simulink model "test2"  (R2019b)
settings: Solver=VariableStepAuto  StartTime=0.0  StopTime=10.0  RelTol=1e-3
libraries: simulink x1
settings Model: Creator=yango  LastModifiedBy=yango

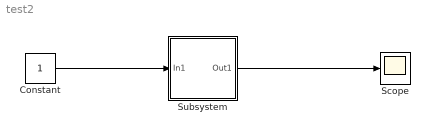
== system test2 ==
  Constant : Constant
  Scope : Scope
  Subsystem : Subsystem
  wires:
  Constant/1 -> Subsystem/1(In1)
  Subsystem/1(Out1) -> Scope/1

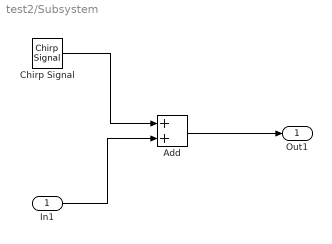
== system test2/Subsystem ==
  In1 : Inport
  Add : Sum
  Chirp Signal : simulink/Sources/Chirp Signal  f1=0.1  T=100  f2=1
  Out1 : Outport
  wires:
  Chirp Signal/1 -> Add/1
  In1/1 -> Add/2
  Add/1 -> Out1/1
